simulink model "sm_backhoe"  (R2021b)
settings: Solver=ode23t  StartTime=0.0  StopTime=60  MaxStep=0.1  RelTol=1e-3  EnableMultiTasking=on
model workspace (MATLAB code in the model file):
  | cylinderGray = [0.6 0.6 0.6];
  | darkOrange = [0.8 0.5 0];
  | glassBlue = [0.2 0.2 1];
  | gray = [0.3 0.3 0.3];
  | orange = [0.8 0.65 0];
  | pistonGray = [0.4 0.4 0.4];
  | tireBlack = [0.1 0.1 0.1];
  | wheelGray = [0.6 0.6 0.6];
  | yellow = [0.8 0.8 0];
  | 
  | rhoGlass = 2500;
  | rhoRubber = 1500;
  | rhoSteel = 7800;
undefined symbols (not defined in the file): sigbuilder_block, X, Y, Z
libraries: sm_lib x161, sm_backhoe_lib x38, nesl_utility x9
(part 2 of 5)

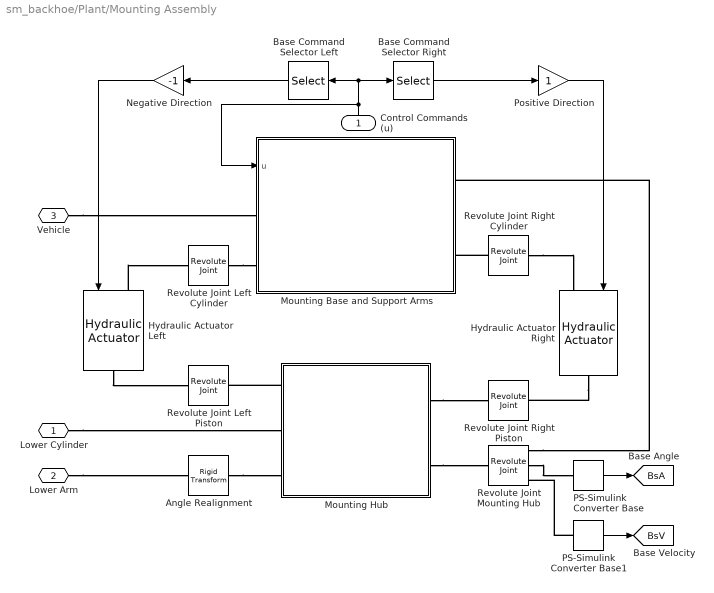
== system sm_backhoe/Plant/Mounting Assembly ==
  Control Commands (u) : Inport
  Angle Realignment : sm_lib/Frames and Transforms/Rigid Transform  TranslationMethod=None  TranslationStandardOffset=0.5  TranslationLengthUnit=m  TranslationStandardAxis=+Z  TranslationCartesianOffset=[ 0 0 0]  TranslationROffset=0  TranslationROffsetUnits=m  TranslationZOffset=0  TranslationZOffsetUnits=m  TranslationThetaOffset=0  TranslationThetaOffsetUnits=deg  RotationMethod=AlignedAxes  RotationAngleUnits=deg  RotationStandardAxis=-Z  RotationAngle=90  RotationArbitraryAxis=[0 0 1]  FollAlignAxisA=+Z  BaseAlignAxisA=+Z  FollAlignAxisB=+X  BaseAlignAxisB=-Y  RotationSequenceAxes=FollowerAxes  RotationSequence=XYX  RotationSequenceAngles=[0 0 0]  RotationSequenceAnglesUnits=deg  RotationMatrix=[1 0 0; 0 1 0; 0 0 1]
  Base Command Selector Left : Selector  InputPortWidth=5  IndexOptions=Index vector (dialog)  Indices=4  OutputSizes=1
  Base Command Selector Right : Selector  InputPortWidth=5  IndexOptions=Index vector (dialog)  Indices=4  OutputSizes=1
  Hydraulic Actuator Left : sm_backhoe_lib/Hydraulic Actuator  Lcyl=1.6  Rcyl=0.15  Lbase=0.65  Wbase=0.35  Rbp=0.075  Lbp=0.8  circlePointsCyl=25  circlePointsCylB=25  Lpist=1.75  Rpist=0.085  Whead=0.275  Lhead=0.5  Rhp=0.075  Lhp=0.9  circlePointsPist=25  cylColor=cylinderGray  rhoCyl=rhoSteel  pistColor=pistonGray  rhoPist=rhoSteel  connColor=gray  rhoConn=rhoSteel
      settings: SourceProductBaseCode=MS
  Hydraulic Actuator Right : sm_backhoe_lib/Hydraulic Actuator  Lcyl=1.6  Rcyl=0.15  Lbase=0.65  Wbase=0.35  Rbp=0.075  Lbp=0.8  circlePointsCyl=25  circlePointsCylB=25  Lpist=1.75  Rpist=0.085  Whead=0.275  Lhead=0.5  Rhp=0.075  Lhp=0.9  circlePointsPist=25  cylColor=cylinderGray  rhoCyl=rhoSteel  pistColor=pistonGray  rhoPist=rhoSteel  connColor=gray  rhoConn=rhoSteel
      settings: SourceProductBaseCode=MS
  Mounting Base and Support Arms : Subsystem
      mask Display:
      | image(fullfile(matlabroot,'toolbox','physmod','sm','smdemos','backhoe','images','sm_backhoe_mountingbaseassembly.png'));
      | port_label('input',1,'u');
      | port_label('lconn',1,'V');
      | port_label('lconn',2,'AL');
      | port_label('rconn',1,'MH');
      | port_label('rconn',2,'AR');
  Mounting Hub : Subsystem  mask(Mounting Hub){Hleft=1, Hright=2, Ltop=0.75, Lbottom=1.5, Tplate=0.3, Dplates=1.2, plateFillet=0.25, numPoints=15, L1=0.75, H1=0.25, RH1=0.075, L2=0.75, H2=1.75, RH2=0.075, L3=0.5, H3=0.5, Larm=0.8, Warm=0.5, Tarm=0.5, Tab=0.1, RH3=0.075, Dbracket=1.1, Lbracket=1.2, Wbracket=1.2, Tbracket=2, Hbracket=1, Rhole=0.1, Hhole=0.5, hubColor=orange, rho=rhoSteel}
      mask prompts: Hleft "Hleft (m)"; Hright "Hright (m)"; Ltop "Ltop (m)"; Lbottom "Lbottom (m)"; Tplate "Tplate (m)"; Dplates "Dplates (m)"; plateFillet "Plate Fillet Radius (m)"; numPoints "Fillet Resolution (pts/rev)"; L1 "L1 (m)"; H1 "H1 (m)"; RH1 "RH1 (m)"; L2 "L2 (m)"; H2 "H2 (m)"; RH2 "RH2 (m)"; L3 "L3 (m)"; H3 "H3 (m)"; Larm "Larm (m)"; Warm "Warm (m)"; Tarm "Tarm (m)"; Tab "Tab (m)"; RH3 "RH3 (m)"; Dbracket "Dbracket (m)"; Lbracket "Lbracket (m)"; Wbracket "Wbracket (m)"; Tbracket "Tbracket (m)"; Hbracket "Hbracket (m)"; Rhole "Rhole (m)"; Hhole "Hhole (m)"; hubColor "Hub Color"; rho "Density (kg/m^3)"
      mask help:
      | Consists of the backhoe mounting hub assembly.
      |
      | This assembly connects to the Backhoe Arm assembly on the front end, and to the Mounting Base assembly on the rear and side.
      |
      | Attachment points are:
      | LH: Left base hydraulic actuator (piston Head).
      | RH: Right base hydraulic actuator (piston Head).
      | LC: Lower arm hydraulic actuator (Cylinder base).
      | LA: Lower Arm joint.
      | MB: Mounting Base joint.
      | All attachments are configured for Revolute Joints.
      |
      | Click on Help to view a schematic of the bracket, its configurable dimension parameters and attachment points (in red).
      mask init:
      | plateSection = [0              0     ; ...
      |                 Lbottom        0     ; ...
      |                 Lbottom        Hright; ...
      |                 (Lbottom-Ltop) Hright; ...
      |                 0              Hleft];
      | plateSection = simmechanics.demohelpers.round_corners(plateSection,1:5,0.1,15);
      mask Help: web(fullfile(matlabroot,'toolbox','physmod','sm','smdemos','backhoe','demohelp','sm_backhoe_mountinghub.html'));
      mask Display:
      | image(fullfile(matlabroot,'toolbox','physmod','sm','smdemos','backhoe','images','sm_backhoe_mountinghub.png'));
      | port_label('lconn',1,'LH');
      | port_label('lconn',2,'LC');
      | port_label('lconn',3,'LA');
      | port_label('rconn',1,'RH');
      | port_label('rconn',2,'MB');
  Negative Direction : Gain  Gain=-1
  PS-Simulink Converter Base : nesl_utility/PS-Simulink Converter  PhysicalDomain=network_engine_domain  SubClassName=ps_output  LeftPortType=input  RightPortType=output  PseudoPeriodic=off  Frequencies=[]  Unit=deg  AffineConversion=off
      settings: SourceProductBaseCode=PW,SS
  PS-Simulink Converter Base1 : nesl_utility/PS-Simulink Converter  PhysicalDomain=network_engine_domain  SubClassName=ps_output  LeftPortType=input  RightPortType=output  PseudoPeriodic=off  Frequencies=[]  Unit=deg/s  AffineConversion=off
      settings: SourceProductBaseCode=PW,SS
  Positive Direction : Gain
  Revolute Joint Left Cylinder : sm_lib/Joints/Revolute Joint  JointMode=Normal  SenseConstraintForce=off  SenseConstraintForceX=off  SenseConstraintForceY=off  SenseConstraintForceZ=off  SenseConstraintTorque=off  SenseConstraintTorqueX=off  SenseConstraintTorqueY=off  SenseConstraintTorqueZ=off  SenseTotalForce=off  SenseTotalForceX=off  SenseTotalForceY=off  SenseTotalForceZ=off  SenseTotalTorque=off  SenseTotalTorqueX=off  SenseTotalTorqueY=off  SenseTotalTorqueZ=off  CompositeWrenchDir=FollowerOnBase  CompositeWrenchFrame=BaseFrame  EquilibriumPosition=0  EquilibriumPositionUnits=deg  SpringStiffness=0  SpringStiffnessUnits=N*m/deg  DampingCoefficient=0  DampingCoefficientUnits=N*m/(deg/s)  TorqueActuationMode=NoTorque  MotionActuationMode=ComputedMotion  SensePosition=off  SenseVelocity=off  SenseAcceleration=off  SenseTorqueForce=off  SenseLowerLimitTorqueForce=off  SenseUpperLimitTorqueForce=off  LowerLimitSpecify=off  LowerLimitBound=-90  LowerLimitBoundUnits=deg  LowerLimitStiffness=1e4  LowerLimitStiffnessUnits=N*m/deg  LowerLimitDamping=10  LowerLimitDampingUnits=N*m/(deg/s)  LowerLimitTransitionRegionWidth=0.1  LowerLimitTransitionRegionWidthUnits=deg  UpperLimitSpecify=off  UpperLimitBound=90  UpperLimitBoundUnits=deg  UpperLimitStiffness=1e4  UpperLimitStiffnessUnits=N*m/deg  UpperLimitDamping=10  UpperLimitDampingUnits=N*m/(deg/s)  UpperLimitTransitionRegionWidth=0.1  UpperLimitTransitionRegionWidthUnits=deg  PositionTargetSpecify=off  PositionTargetPriority=High  PositionTargetValue=0  PositionTargetValueUnits=deg  VelocityTargetSpecify=off  VelocityTargetPriority=High  VelocityTargetValue=0  VelocityTargetValueUnits=deg/s
  Revolute Joint Right Cylinder : sm_lib/Joints/Revolute Joint  JointMode=Normal  SenseConstraintForce=off  SenseConstraintForceX=off  SenseConstraintForceY=off  SenseConstraintForceZ=off  SenseConstraintTorque=off  SenseConstraintTorqueX=off  SenseConstraintTorqueY=off  SenseConstraintTorqueZ=off  SenseTotalForce=off  SenseTotalForceX=off  SenseTotalForceY=off  SenseTotalForceZ=off  SenseTotalTorque=off  SenseTotalTorqueX=off  SenseTotalTorqueY=off  SenseTotalTorqueZ=off  CompositeWrenchDir=FollowerOnBase  CompositeWrenchFrame=BaseFrame  EquilibriumPosition=0  EquilibriumPositionUnits=deg  SpringStiffness=0  SpringStiffnessUnits=N*m/deg  DampingCoefficient=0  DampingCoefficientUnits=N*m/(deg/s)  TorqueActuationMode=NoTorque  MotionActuationMode=ComputedMotion  SensePosition=off  SenseVelocity=off  SenseAcceleration=off  SenseTorqueForce=off  SenseLowerLimitTorqueForce=off  SenseUpperLimitTorqueForce=off  LowerLimitSpecify=off  LowerLimitBound=-90  LowerLimitBoundUnits=deg  LowerLimitStiffness=1e4  LowerLimitStiffnessUnits=N*m/deg  LowerLimitDamping=10  LowerLimitDampingUnits=N*m/(deg/s)  LowerLimitTransitionRegionWidth=0.1  LowerLimitTransitionRegionWidthUnits=deg  UpperLimitSpecify=off  UpperLimitBound=90  UpperLimitBoundUnits=deg  UpperLimitStiffness=1e4  UpperLimitStiffnessUnits=N*m/deg  UpperLimitDamping=10  UpperLimitDampingUnits=N*m/(deg/s)  UpperLimitTransitionRegionWidth=0.1  UpperLimitTransitionRegionWidthUnits=deg  PositionTargetSpecify=off  PositionTargetPriority=High  PositionTargetValue=0  PositionTargetValueUnits=deg  VelocityTargetSpecify=off  VelocityTargetPriority=High  VelocityTargetValue=0  VelocityTargetValueUnits=deg/s
  Revolute Joint Mounting Hub : sm_lib/Joints/Revolute Joint  JointMode=Normal  SenseConstraintForce=off  SenseConstraintForceX=off  SenseConstraintForceY=off  SenseConstraintForceZ=off  SenseConstraintTorque=off  SenseConstraintTorqueX=off  SenseConstraintTorqueY=off  SenseConstraintTorqueZ=off  SenseTotalForce=off  SenseTotalForceX=off  SenseTotalForceY=off  SenseTotalForceZ=off  SenseTotalTorque=off  SenseTotalTorqueX=off  SenseTotalTorqueY=off  SenseTotalTorqueZ=off  CompositeWrenchDir=FollowerOnBase  CompositeWrenchFrame=BaseFrame  EquilibriumPosition=0  EquilibriumPositionUnits=deg  SpringStiffness=1000  SpringStiffnessUnits=N*m/rad  DampingCoefficient=500  DampingCoefficientUnits=N*m/(rad/s)  TorqueActuationMode=NoTorque  MotionActuationMode=ComputedMotion  SensePosition=on  SenseVelocity=on  SenseAcceleration=off  SenseTorqueForce=off  SenseLowerLimitTorqueForce=off  SenseUpperLimitTorqueForce=off  LowerLimitSpecify=off  LowerLimitBound=-90  LowerLimitBoundUnits=deg  LowerLimitStiffness=1e4  LowerLimitStiffnessUnits=N*m/deg  LowerLimitDamping=10  LowerLimitDampingUnits=N*m/(deg/s)  LowerLimitTransitionRegionWidth=0.1  LowerLimitTransitionRegionWidthUnits=deg  UpperLimitSpecify=off  UpperLimitBound=90  UpperLimitBoundUnits=deg  UpperLimitStiffness=1e4  UpperLimitStiffnessUnits=N*m/deg  UpperLimitDamping=10  UpperLimitDampingUnits=N*m/(deg/s)  UpperLimitTransitionRegionWidth=0.1  UpperLimitTransitionRegionWidthUnits=deg  PositionTargetSpecify=on  PositionTargetPriority=Low  PositionTargetValue=0  PositionTargetValueUnits=deg  VelocityTargetSpecify=off  VelocityTargetPriority=High  VelocityTargetValue=0  VelocityTargetValueUnits=deg/s
  Revolute Joint Left Piston : sm_lib/Joints/Revolute Joint  JointMode=Normal  SenseConstraintForce=off  SenseConstraintForceX=off  SenseConstraintForceY=off  SenseConstraintForceZ=off  SenseConstraintTorque=off  SenseConstraintTorqueX=off  SenseConstraintTorqueY=off  SenseConstraintTorqueZ=off  SenseTotalForce=off  SenseTotalForceX=off  SenseTotalForceY=off  SenseTotalForceZ=off  SenseTotalTorque=off  SenseTotalTorqueX=off  SenseTotalTorqueY=off  SenseTotalTorqueZ=off  CompositeWrenchDir=FollowerOnBase  CompositeWrenchFrame=BaseFrame  EquilibriumPosition=0  EquilibriumPositionUnits=deg  SpringStiffness=0  SpringStiffnessUnits=N*m/deg  DampingCoefficient=0  DampingCoefficientUnits=N*m/(deg/s)  TorqueActuationMode=NoTorque  MotionActuationMode=ComputedMotion  SensePosition=off  SenseVelocity=off  SenseAcceleration=off  SenseTorqueForce=off  SenseLowerLimitTorqueForce=off  SenseUpperLimitTorqueForce=off  LowerLimitSpecify=off  LowerLimitBound=-90  LowerLimitBoundUnits=deg  LowerLimitStiffness=1e4  LowerLimitStiffnessUnits=N*m/deg  LowerLimitDamping=10  LowerLimitDampingUnits=N*m/(deg/s)  LowerLimitTransitionRegionWidth=0.1  LowerLimitTransitionRegionWidthUnits=deg  UpperLimitSpecify=off  UpperLimitBound=90  UpperLimitBoundUnits=deg  UpperLimitStiffness=1e4  UpperLimitStiffnessUnits=N*m/deg  UpperLimitDamping=10  UpperLimitDampingUnits=N*m/(deg/s)  UpperLimitTransitionRegionWidth=0.1  UpperLimitTransitionRegionWidthUnits=deg  PositionTargetSpecify=off  PositionTargetPriority=Low  PositionTargetValue=180  PositionTargetValueUnits=deg  VelocityTargetSpecify=off  VelocityTargetPriority=High  VelocityTargetValue=0  VelocityTargetValueUnits=deg/s
  Revolute Joint Right Piston : sm_lib/Joints/Revolute Joint  JointMode=Normal  SenseConstraintForce=off  SenseConstraintForceX=off  SenseConstraintForceY=off  SenseConstraintForceZ=off  SenseConstraintTorque=off  SenseConstraintTorqueX=off  SenseConstraintTorqueY=off  SenseConstraintTorqueZ=off  SenseTotalForce=off  SenseTotalForceX=off  SenseTotalForceY=off  SenseTotalForceZ=off  SenseTotalTorque=off  SenseTotalTorqueX=off  SenseTotalTorqueY=off  SenseTotalTorqueZ=off  CompositeWrenchDir=FollowerOnBase  CompositeWrenchFrame=BaseFrame  EquilibriumPosition=0  EquilibriumPositionUnits=deg  SpringStiffness=0  SpringStiffnessUnits=N*m/deg  DampingCoefficient=0  DampingCoefficientUnits=N*m/(deg/s)  TorqueActuationMode=NoTorque  MotionActuationMode=ComputedMotion  SensePosition=off  SenseVelocity=off  SenseAcceleration=off  SenseTorqueForce=off  SenseLowerLimitTorqueForce=off  SenseUpperLimitTorqueForce=off  LowerLimitSpecify=off  LowerLimitBound=-90  LowerLimitBoundUnits=deg  LowerLimitStiffness=1e4  LowerLimitStiffnessUnits=N*m/deg  LowerLimitDamping=10  LowerLimitDampingUnits=N*m/(deg/s)  LowerLimitTransitionRegionWidth=0.1  LowerLimitTransitionRegionWidthUnits=deg  UpperLimitSpecify=off  UpperLimitBound=90  UpperLimitBoundUnits=deg  UpperLimitStiffness=1e4  UpperLimitStiffnessUnits=N*m/deg  UpperLimitDamping=10  UpperLimitDampingUnits=N*m/(deg/s)  UpperLimitTransitionRegionWidth=0.1  UpperLimitTransitionRegionWidthUnits=deg  PositionTargetSpecify=off  PositionTargetPriority=Low  PositionTargetValue=0  PositionTargetValueUnits=deg  VelocityTargetSpecify=off  VelocityTargetPriority=High  VelocityTargetValue=0  VelocityTargetValueUnits=deg/s
  Lower Cylinder : PMIOPort  Side=Right
  Lower Arm : PMIOPort  Port=2  Side=Right
  Vehicle : PMIOPort  Port=3  Side=Left
  tag scope: BsA=global, BsV=global
  wires:
  Control Commands (u)/1 -> Base Command Selector Left/1, Base Command Selector Right/1, Mounting Base and Support Arms/1(u)
  PS-Simulink Converter Base/1 -> [BsA]
  Base Command Selector Left/1 -> Negative Direction/1
  Base Command Selector Right/1 -> Positive Direction/1
  Negative Direction/1 -> Hydraulic Actuator Left/1
  Positive Direction/1 -> Hydraulic Actuator Right/1
  PS-Simulink Converter Base1/1 -> [BsV]
  connections:
  Mounting Hub/RConn2 -- Revolute Joint Mounting Hub/LConn1
  Mounting Hub/LConn1 -- Revolute Joint Left Piston/RConn1
  Mounting Hub/RConn1 -- Revolute Joint Right Piston/RConn1
  Vehicle/RConn1 -- Mounting Base and Support Arms/LConn1
  Revolute Joint Mounting Hub/RConn1 -- Mounting Base and Support Arms/RConn1
  Revolute Joint Mounting Hub/RConn2 -- PS-Simulink Converter Base/LConn1
  Lower Arm/RConn1 -- Angle Realignment/RConn1
  Angle Realignment/LConn1 -- Mounting Hub/LConn3
  Revolute Joint Left Cylinder/LConn1 -- Mounting Base and Support Arms/LConn2
  Revolute Joint Right Cylinder/LConn1 -- Mounting Base and Support Arms/RConn2
  Revolute Joint Right Cylinder/RConn1 -- Hydraulic Actuator Right/LConn1
  Hydraulic Actuator Right/RConn1 -- Revolute Joint Right Piston/LConn1
  Hydraulic Actuator Left/RConn1 -- Revolute Joint Left Piston/LConn1
  Hydraulic Actuator Left/LConn1 -- Revolute Joint Left Cylinder/RConn1
  Lower Cylinder/RConn1 -- Mounting Hub/LConn2
  PS-Simulink Converter Base1/LConn1 -- Revolute Joint Mounting Hub/RConn3

== system sm_backhoe/Plant/Sensed Signals ==
  Vector Concatenate : Concatenate  NumInputs=10
  pv : Outport
  wires:
  [BuA] -> Vector Concatenate/1
  [SV] -> Vector Concatenate/10
  [SA] -> Vector Concatenate/9
  [BsV] -> Vector Concatenate/8
  [BsA] -> Vector Concatenate/7
  [LV] -> Vector Concatenate/6
  [LA] -> Vector Concatenate/5
  [UV] -> Vector Concatenate/4
  [UA] -> Vector Concatenate/3
  [BuV] -> Vector Concatenate/2
  Vector Concatenate/1 -> pv/1

== system sm_backhoe/Plant/Vehicle ==
  " Rear Right Wheel" : sm_backhoe_lib/Wheel  Rwheel=1  Rtire=1.75  Raxle=0.15  W=1.65  Nc=30  tireColor=tireBlack  rhoTire=rhoRubber  wheelColor=wheelGray  rhoWheel=rhoSteel
      settings: SourceProductBaseCode=MS
  Front Left Wheel : sm_backhoe_lib/Wheel  Rwheel=0.85  Rtire=1.5  Raxle=0.15  W=1.2  Nc=30  tireColor=tireBlack  rhoTire=rhoRubber  wheelColor=wheelGray  rhoWheel=rhoSteel
      settings: SourceProductBaseCode=MS
  Front Right Wheel : sm_backhoe_lib/Wheel  Rwheel=0.85  Rtire=1.5  Raxle=0.15  W=1.2  Nc=30  tireColor=tireBlack  rhoTire=rhoRubber  wheelColor=wheelGray  rhoWheel=rhoSteel
      settings: SourceProductBaseCode=MS
  Lower Vehicle : Subsystem  mask(Lower Vehicle){Wbody=3, Lbody=7.75, Hbody=2.25, Lfw=6, Hfw=0.5, Pfw=1.5, Lrw=1.85, Hrw=0.75, Prw=2, Raxle=0.15, color=yellow, rho=rhoSteel}
      mask prompts: Wbody "Wbody (m)"; Lbody "Lbody (m)"; Hbody "Hbody (m)"; Lfw "Lfw (m)"; Hfw "Hfw (m)"; Pfw "Pfw (m)"; Lrw "Lrw (m)"; Hrw "Hrw (m)"; Prw "Prw (m)"; Raxle "Raxle (m)"; color "Chassis Color"; rho "Density (kg/m^3)"
      mask help:
      | Consists of the backhoe lower vehicle assembly.
      |
      | Rigid attachment points are:
      | MA: Mounting Assembly.
      | UV: Upper Vehicle.
      |
      | Revolute joint attachment points are:
      | FLW: Front Left Wheel.
      | RLW: Rear Left Wheel.
      | FRW: Front Right Wheel.
      | RRW: Rear Right Wheel.
      |
      | Click on Help to view a schematic of the lower vehicle, its configurable dimension parameters and attachment points (in red).
      mask Help: web(fullfile(matlabroot,'toolbox','physmod','sm','smdemos','backhoe','demohelp','sm_backhoe_lowervehicle.html'));
      mask Display:
      | image(fullfile(matlabroot,'toolbox','physmod','sm','smdemos','backhoe','images','sm_backhoe_lowervehicle.png'));
      | port_label('rconn',1,'MA');
      | port_label('lconn',2,'RRW');
      | port_label('lconn',3,'FRW');
      | port_label('lconn',1,'UV');
      | port_label('rconn',2,'RLW');
      | port_label('rconn',3,'FLW');
  Rear Left Wheel : sm_backhoe_lib/Wheel  Rwheel=1  Rtire=1.75  Raxle=0.15  W=1.65  Nc=30  tireColor=tireBlack  rhoTire=rhoRubber  wheelColor=wheelGray  rhoWheel=rhoSteel
      settings: SourceProductBaseCode=MS
  Upper Vehicle : Subsystem  mask(Upper Vehicle){D=-0.25, L1=3.5, L2=2.5, L3=2, L4=1.5, H=4, W=2.75, T=0.2, Wroof=3.75, Lroof=4.4, Troof=0.4, Rfillet=0.75, numPoints=25, Hback=1.5, Wback=3, Lback=1.52, backFillet=1, roofColor=yellow, rhoRoof=rhoSteel, cageColor=gray, rhoCage=rhoSteel, windowColor=glassBlue, rhoWindow=rhoGlass, opacity=0.6, backColor=yellow, rhoBack=rhoSteel}
      mask prompts: D "D (m)"; L1 "L1 (m)"; L2 "L2 (m)"; L3 "L3 (m)"; L4 "L4 (m)"; H "H (m)"; W "W (m)"; T "T (m)"; Wroof "Wroof (m)"; Lroof "Lroof (m)"; Troof "Troof (m)"; Rfillet "Rfillet [m]"; numPoints "Fillet Point Resolution"; Hback "Hback (m)"; Wback "Wback (m)"; Lback "Lback (m)"; backFillet "backFillet (m)"; roofColor "Roof Color"; rhoRoof "Roof Density (kg/m^3)"; cageColor "Cage Color"; rhoCage "Cage Density (kg/m^3)"; windowColor "Window Color"; rhoWindow "Window Density (kg/m^3)"; opacity "Window Opacity"; backColor "Back Color"; rhoBack "Back Density (kg/m^3)"
      mask help:
      | Consists of the backhoe upper vehicle assembly. Components are the glass cage, the back and the roof of the backhoe model.
      |
      | There is one rigid attachment points to the Lower Vehicle (LV).
      |
      | Click on Help to view a schematic of the upper vehicle, its configurable dimension parameters and attachment points (in red).
      mask init:
      | fWindow = [-T/2          0.01 ; ...
      |            -T/2          H    ; ...
      |            -L3           H    ; ...
      |            -(L1-T/2)     0.01];
      |        
      | bWindow = [T/2          0.01 ; ...
      |            (L2-T/2)     0.01 ; ...
      |            L4           H    ; ...
      |            T/2          H   ];
      | 
      | roofSection = [ Wroof/2  Lroof/2; ...
      |                -Wroof/2  Lroof/2; ...
      |                -Wroof/2 -Lroof/2; ...
      |                 Wroof/2 -Lroof/2];
      | roofSection = simmechanics.demohelpers.round_corners(roofSection,1:4,Rfillet,numPoints);
      | 
      | theta = atan((L2-L4)/H);
      | 
      | backSection = [  0                     0    ; ...
      |                Lback                   0    ; ...
      |            (Lback-(Hback*sin(theta))) Hback ; ...
      |             -Hback*sin(theta)         Hback];
      | backSection = simmechanics.demohelpers.round_corners(backSection,3,backFillet,numPoints);
      mask Help: web(fullfile(matlabroot,'toolbox','physmod','sm','smdemos','backhoe','demohelp','sm_backhoe_uppervehicle.html'));
      mask Display:
      | image(fullfile(matlabroot,'toolbox','physmod','sm','smdemos','backhoe','images','sm_backhoe_uppervehicle.png'));
      | port_label('lconn',1,'LV');
  Mounting Assembly : PMIOPort  Side=Left
  Ground : PMIOPort  Port=2  Side=Right
  connections:
  Lower Vehicle/RConn1 -- Mounting Assembly/RConn1
  Lower Vehicle/LConn2 -- " Rear Right Wheel"/LConn1
  Lower Vehicle/LConn3 -- Front Right Wheel/LConn1
  Lower Vehicle/RConn3 -- Front Left Wheel/LConn1
  Lower Vehicle/RConn2 -- Rear Left Wheel/LConn1
  Lower Vehicle/LConn1 -- Ground/RConn1 -- Upper Vehicle/LConn1

== system sm_backhoe/Plant/Backhoe Arm/Bucket ==
  Arm Revolute Rotation : sm_lib/Frames and Transforms/Rigid Transform  TranslationMethod=None  TranslationStandardOffset=0  TranslationLengthUnit=m  TranslationStandardAxis=+X  TranslationCartesianOffset=[0 0 0]  TranslationROffset=0  TranslationROffsetUnits=m  TranslationZOffset=0  TranslationZOffsetUnits=m  TranslationThetaOffset=0  TranslationThetaOffsetUnits=deg  RotationMethod=AlignedAxes  RotationAngleUnits=deg  RotationStandardAxis=-Y  RotationAngle=180  RotationArbitraryAxis=[0 0 1]  FollAlignAxisA=+Y  BaseAlignAxisA=+Y  FollAlignAxisB=+X  BaseAlignAxisB=-X  RotationSequenceAxes=FollowerAxes  RotationSequence=XYX  RotationSequenceAngles=[0 0 0]  RotationSequenceAnglesUnits=deg  RotationMatrix=[1 0 0; 0 1 0; 0 0 1]
  Attachment Frame : Subsystem
      mask Display:
      | image(fullfile(matlabroot,'toolbox','physmod','sm','smdemos','backhoe','images','sm_backhoe_attach.png'));
      | port_label('lconn',1,'B');
      | port_label('rconn',1,'CA');
      | port_label('rconn',2,'UA');
  Bucket : Subsystem
      mask Display:
      | image(fullfile(matlabroot,'toolbox','physmod','sm','smdemos','backhoe','images','sm_backhoe_bucketcase.png'));
      | port_label('rconn',1,'AF');
  Crank Revolute Rotation : sm_lib/Frames and Transforms/Rigid Transform  TranslationMethod=None  TranslationStandardOffset=0  TranslationLengthUnit=m  TranslationStandardAxis=+X  TranslationCartesianOffset=[0 0 0]  TranslationROffset=0  TranslationROffsetUnits=m  TranslationZOffset=0  TranslationZOffsetUnits=m  TranslationThetaOffset=0  TranslationThetaOffsetUnits=deg  RotationMethod=AlignedAxes  RotationAngleUnits=deg  RotationStandardAxis=-Y  RotationAngle=180  RotationArbitraryAxis=[0 0 1]  FollAlignAxisA=+Y  BaseAlignAxisA=+Y  FollAlignAxisB=+X  BaseAlignAxisB=-X  RotationSequenceAxes=FollowerAxes  RotationSequence=XYX  RotationSequenceAngles=[0 0 0]  RotationSequenceAnglesUnits=deg  RotationMatrix=[1 0 0; 0 1 0; 0 0 1]
  Crank Arm : PMIOPort  Side=Right
  Upper Arm : PMIOPort  Port=2  Side=Right
  connections:
  Bucket/RConn1 -- Attachment Frame/LConn1
  Crank Revolute Rotation/LConn1 -- Attachment Frame/RConn1
  Arm Revolute Rotation/LConn1 -- Attachment Frame/RConn2
  Upper Arm/RConn1 -- Arm Revolute Rotation/RConn1
  Crank Arm/RConn1 -- Crank Revolute Rotation/RConn1

== system sm_backhoe/Plant/Backhoe Arm/Lower Arm Assembly ==
  Angle Rotation : sm_lib/Frames and Transforms/Rigid Transform  TranslationMethod=None  TranslationStandardOffset=0  TranslationLengthUnit=m  TranslationStandardAxis=+Z  TranslationCartesianOffset=[0 0 0]  TranslationROffset=0  TranslationROffsetUnits=m  TranslationZOffset=0  TranslationZOffsetUnits=m  TranslationThetaOffset=0  TranslationThetaOffsetUnits=deg  RotationMethod=AlignedAxes  RotationAngleUnits=deg  RotationStandardAxis=+Z  RotationAngle=180  RotationArbitraryAxis=[0 0 1]  FollAlignAxisA=+Z  BaseAlignAxisA=+Z  FollAlignAxisB=+Y  BaseAlignAxisB=-Y  RotationSequenceAxes=FollowerAxes  RotationSequence=XYX  RotationSequenceAngles=[0 0 0]  RotationSequenceAnglesUnits=deg  RotationMatrix=[1 0 0; 0 1 0; 0 0 1]
  Bracket Double Hole : sm_backhoe_lib/Bracket Double Hole  Hbracket=0.75  Wbracket=1.5  Tbracket=0.15  Dbracket=0.75  Hhole=0.5  Dhole=0.75  Rhole=0.075  Rfillet=0.375  Nc=25  bracketColor=orange  rho=rhoSteel
      settings: SourceProductBaseCode=MS
  Front Bracket : sm_backhoe_lib/Bracket  Hbracket=0.65  Wbracket=0.5  Tbracket=0.225  Dbracket=0.45  Hhole=0.4  Rhole=0.075  circlePoints=25  bracketColor=darkOrange  rho=rhoSteel
      settings: SourceProductBaseCode=MS
  Lower Arm : Subsystem  mask(Lower Arm){Lbar=7, Wbar=0.8, Tbar=0.85, Lb=0.5, barFillet=0.1, numPoints=15, armColor=yellow, rho=rhoSteel}
      mask prompts: Lbar "Lbar (m)"; Wbar "Wbar (m)"; Tbar "Tbar (m)"; Lb "Lb (m)"; barFillet "Bar Fillet Radius (m)"; numPoints "Fillet Resolution (pts/rev)"; armColor "Arm Color"; rho "Density (kg/m^3)"
      mask help:
      | Consists of the backhoe lower arm and three attachment brackets -- front, rear and upper
      |
      | Attachment Points are:
      | MA: Mounting Assembly attachment.
      | LH: Lower arm hydraulic actuator (piston Head).
      | UA: Upper arm attachment.
      | UC: Upper arm hydraulic actuator (Cylinder base).
      | All attachments are configured for Revolute joints.
      |
      | The length Lb corresponds to the lengths measured from the center of the bar to the center of the upper bracket.
      |
      | The front and rear brackets are automatically placed at the center of the end faces of the upper arm bar.
      |
      | Click on Help to view a schematic of the lower arm, its configurable dimension parameters and attachment points (in red).
      mask init:
      | barSection = [Tbar/2 Wbar/2;  ...
      |              -Tbar/2 Wbar/2;  ...
      |              -Tbar/2 -Wbar/2; ...
      |               Tbar/2 -Wbar/2];
      | barSection = simmechanics.demohelpers.round_corners(barSection,1:4,barFillet,numPoints);
      mask Help: web(fullfile(matlabroot,'toolbox','physmod','sm','smdemos','backhoe','demohelp','sm_backhoe_lowerarm.html'));
      mask Display:
      | image(fullfile(matlabroot,'toolbox','physmod','sm','smdemos','backhoe','images','sm_backhoe_lowerarm.png'));
      | port_label('rconn',1,'RB');
      | port_label('lconn',2,'FB');;
      | port_label('lconn',1,'UB');
  Pin : sm_lib/Body Elements/Cylindrical Solid  GraphicAmbientColor=[0.15 0.15 0.15 1.0]  BasedOnType=Density  CenterOfMass=[0 0 0]  CenterOfMassUnits=m  GraphicDiffuseColor=gray  CylinderLength=0.8  CylinderLengthUnits=m  CylinderRadius=0.075  CylinderRadiusUnits=m  Density=rhoSteel  DensityUnits=kg/(m^3)  DoExposeReferenceFrame=on  GraphicEmissiveColor=[0.0 0.0 0.0 1.0]  ExportEntireGeometry=off  SerializedFrames=<Frames/>  MarkerShape=Sphere  MarkerSize=10  GraphicType=FromGeometry  InertiaType=CalculateFromGeometry  Mass=1  MassUnits=kg  MomentsOfInertia=[1 1 1]  MomentsOfInertiaUnits=kg*m^2  GraphicOpacity=1.0  ProductsOfInertia=[0 0 0]  ProductsOfInertiaUnits=kg*m^2  GraphicShininess=75  GraphicSpecularColor=[0.5 0.5 0.5 1.0]  GraphicVisPropType=SimpleVisualProperties
  Pin1 : sm_lib/Body Elements/Cylindrical Solid  GraphicAmbientColor=[0.15 0.15 0.15 1.0]  BasedOnType=Density  CenterOfMass=[0 0 0]  CenterOfMassUnits=m  GraphicDiffuseColor=gray  CylinderLength=0.8  CylinderLengthUnits=m  CylinderRadius=0.075  CylinderRadiusUnits=m  Density=rhoSteel  DensityUnits=kg/(m^3)  DoExposeReferenceFrame=on  GraphicEmissiveColor=[0.0 0.0 0.0 1.0]  ExportEntireGeometry=off  SerializedFrames=<Frames/>  MarkerShape=Sphere  MarkerSize=10  GraphicType=FromGeometry  InertiaType=CalculateFromGeometry  Mass=1  MassUnits=kg  MomentsOfInertia=[1 1 1]  MomentsOfInertiaUnits=kg*m^2  GraphicOpacity=1.0  ProductsOfInertia=[0 0 0]  ProductsOfInertiaUnits=kg*m^2  GraphicShininess=75  GraphicSpecularColor=[0.5 0.5 0.5 1.0]  GraphicVisPropType=SimpleVisualProperties
  Pin2 : sm_lib/Body Elements/Cylindrical Solid  GraphicAmbientColor=[0.15 0.15 0.15 1.0]  BasedOnType=Density  CenterOfMass=[0 0 0]  CenterOfMassUnits=m  GraphicDiffuseColor=gray  CylinderLength=0.8  CylinderLengthUnits=m  CylinderRadius=0.075  CylinderRadiusUnits=m  Density=rhoSteel  DensityUnits=kg/(m^3)  DoExposeReferenceFrame=on  GraphicEmissiveColor=[0.0 0.0 0.0 1.0]  ExportEntireGeometry=off  SerializedFrames=<Frames/>  MarkerShape=Sphere  MarkerSize=10  GraphicType=FromGeometry  InertiaType=CalculateFromGeometry  Mass=1  MassUnits=kg  MomentsOfInertia=[1 1 1]  MomentsOfInertiaUnits=kg*m^2  GraphicOpacity=1.0  ProductsOfInertia=[0 0 0]  ProductsOfInertiaUnits=kg*m^2  GraphicShininess=75  GraphicSpecularColor=[0.5 0.5 0.5 1.0]  GraphicVisPropType=SimpleVisualProperties
  Rear Bracket : sm_backhoe_lib/Bracket  Hbracket=0.75  Wbracket=0.75  Tbracket=0.15  Dbracket=0.75  Hhole=0.5  Rhole=0.075  circlePoints=25  bracketColor=darkOrange  rho=rhoSteel
      settings: SourceProductBaseCode=MS
  Lower Head : PMIOPort  Side=Left
  Mounting Assembly : PMIOPort  Port=2  Side=Left
  Upper Cylinder : PMIOPort  Port=3  Side=Right
  Upper Arm : PMIOPort  Port=4  Side=Right
  connections:
  Mounting Assembly/RConn1 -- Rear Bracket/RConn1
  Lower Arm/RConn1 -- Rear Bracket/LConn1
  Front Bracket/RConn1 -- Pin/RConn1 -- Angle Rotation/LConn1
  Front Bracket/LConn1 -- Lower Arm/LConn2
  Upper Arm/RConn1 -- Angle Rotation/RConn1
  Lower Arm/LConn1 -- Bracket Double Hole/LConn1
  Lower Head/RConn1 -- Bracket Double Hole/RConn2 -- Pin1/RConn1
  Pin2/RConn1 -- Bracket Double Hole/RConn1 -- Upper Cylinder/RConn1

== system sm_backhoe/Plant/Backhoe Arm/Upper Arm Assembly ==
  Pressure [Bucket Joint] : Inport
  Angle Realignment : sm_lib/Frames and Transforms/Rigid Transform  TranslationMethod=None  TranslationStandardOffset=0  TranslationLengthUnit=m  TranslationStandardAxis=+Z  TranslationCartesianOffset=[0 0 0]  TranslationROffset=0  TranslationROffsetUnits=m  TranslationZOffset=0  TranslationZOffsetUnits=m  TranslationThetaOffset=0  TranslationThetaOffsetUnits=deg  RotationMethod=AlignedAxes  RotationAngleUnits=deg  RotationStandardAxis=-Z  RotationAngle=90  RotationArbitraryAxis=[0 0 1]  FollAlignAxisA=+X  BaseAlignAxisA=-Y  FollAlignAxisB=+Z  BaseAlignAxisB=+Z  RotationSequenceAxes=FollowerAxes  RotationSequence=XYX  RotationSequenceAngles=[0 0 0]  RotationSequenceAnglesUnits=deg  RotationMatrix=[1 0 0; 0 1 0; 0 0 1]
  Arm-Actuator Joint : sm_lib/Joints/Revolute Joint  JointMode=Normal  SenseConstraintForce=off  SenseConstraintForceX=off  SenseConstraintForceY=off  SenseConstraintForceZ=off  SenseConstraintTorque=off  SenseConstraintTorqueX=off  SenseConstraintTorqueY=off  SenseConstraintTorqueZ=off  SenseTotalForce=off  SenseTotalForceX=off  SenseTotalForceY=off  SenseTotalForceZ=off  SenseTotalTorque=off  SenseTotalTorqueX=off  SenseTotalTorqueY=off  SenseTotalTorqueZ=off  CompositeWrenchDir=FollowerOnBase  CompositeWrenchFrame=BaseFrame  EquilibriumPosition=0  EquilibriumPositionUnits=deg  SpringStiffness=0  SpringStiffnessUnits=N*m/deg  DampingCoefficient=0  DampingCoefficientUnits=N*m/(deg/s)  TorqueActuationMode=NoTorque  MotionActuationMode=ComputedMotion  SensePosition=off  SenseVelocity=off  SenseAcceleration=off  SenseTorqueForce=off  SenseLowerLimitTorqueForce=off  SenseUpperLimitTorqueForce=off  LowerLimitSpecify=off  LowerLimitBound=-90  LowerLimitBoundUnits=deg  LowerLimitStiffness=1e4  LowerLimitStiffnessUnits=N*m/deg  LowerLimitDamping=10  LowerLimitDampingUnits=N*m/(deg/s)  LowerLimitTransitionRegionWidth=0.1  LowerLimitTransitionRegionWidthUnits=deg  UpperLimitSpecify=off  UpperLimitBound=90  UpperLimitBoundUnits=deg  UpperLimitStiffness=1e4  UpperLimitStiffnessUnits=N*m/deg  UpperLimitDamping=10  UpperLimitDampingUnits=N*m/(deg/s)  UpperLimitTransitionRegionWidth=0.1  UpperLimitTransitionRegionWidthUnits=deg  PositionTargetSpecify=on  PositionTargetPriority=Low  PositionTargetValue=-90  PositionTargetValueUnits=deg  VelocityTargetSpecify=off  VelocityTargetPriority=High  VelocityTargetValue=0  VelocityTargetValueUnits=deg/s
  Crank-Actuator Joint : sm_lib/Joints/Revolute Joint  JointMode=Normal  SenseConstraintForce=off  SenseConstraintForceX=off  SenseConstraintForceY=off  SenseConstraintForceZ=off  SenseConstraintTorque=off  SenseConstraintTorqueX=off  SenseConstraintTorqueY=off  SenseConstraintTorqueZ=off  SenseTotalForce=off  SenseTotalForceX=off  SenseTotalForceY=off  SenseTotalForceZ=off  SenseTotalTorque=off  SenseTotalTorqueX=off  SenseTotalTorqueY=off  SenseTotalTorqueZ=off  CompositeWrenchDir=FollowerOnBase  CompositeWrenchFrame=BaseFrame  EquilibriumPosition=0  EquilibriumPositionUnits=deg  SpringStiffness=0  SpringStiffnessUnits=N*m/deg  DampingCoefficient=0  DampingCoefficientUnits=N*m/(deg/s)  TorqueActuationMode=NoTorque  MotionActuationMode=ComputedMotion  SensePosition=off  SenseVelocity=off  SenseAcceleration=off  SenseTorqueForce=off  SenseLowerLimitTorqueForce=off  SenseUpperLimitTorqueForce=off  LowerLimitSpecify=off  LowerLimitBound=-90  LowerLimitBoundUnits=deg  LowerLimitStiffness=1e4  LowerLimitStiffnessUnits=N*m/deg  LowerLimitDamping=10  LowerLimitDampingUnits=N*m/(deg/s)  LowerLimitTransitionRegionWidth=0.1  LowerLimitTransitionRegionWidthUnits=deg  UpperLimitSpecify=off  UpperLimitBound=90  UpperLimitBoundUnits=deg  UpperLimitStiffness=1e4  UpperLimitStiffnessUnits=N*m/deg  UpperLimitDamping=10  UpperLimitDampingUnits=N*m/(deg/s)  UpperLimitTransitionRegionWidth=0.1  UpperLimitTransitionRegionWidthUnits=deg  PositionTargetSpecify=off  PositionTargetPriority=High  PositionTargetValue=0  PositionTargetValueUnits=deg  VelocityTargetSpecify=off  VelocityTargetPriority=High  VelocityTargetValue=0  VelocityTargetValueUnits=deg/s
  Hydraulic Actuator Upper Arm - Bucket : sm_backhoe_lib/Hydraulic Actuator  Lcyl=1.9  Rcyl=0.2  Lbase=0.65  Wbase=0.425  Rbp=0.075  Lbp=0.8  circlePointsCyl=25  circlePointsCylB=25  Lpist=1.9  Rpist=0.12  Whead=0.35  Lhead=0.65  Rhp=0.075  Lhp=0.9  circlePointsPist=25  cylColor=cylinderGray  rhoCyl=rhoSteel  pistColor=pistonGray  rhoPist=rhoSteel  connColor=gray  rhoConn=rhoSteel
      settings: SourceProductBaseCode=MS
  Upper Arm and Crank : Subsystem
      mask Display:
      | image(fullfile(matlabroot,'toolbox','physmod','sm','smdemos','backhoe','images','sm_backhoe_upperassembly.png'));
      | port_label('lconn',1,'CB');
      | port_label('lconn',2,'UH');
      | port_label('lconn',3,'LA');
      | port_label('rconn',1,'BA');
      | port_label('rconn',2,'BC');
      | port_label('rconn',3,'BH');
  Upper Head : PMIOPort  Side=Left
  Lower Arm : PMIOPort  Port=2  Side=Left
  Crank Arm : PMIOPort  Port=3  Side=Right
  Bucket : PMIOPort  Port=4  Side=Right
  wires:
  Pressure [Bucket Joint]/1 -> Hydraulic Actuator Upper Arm - Bucket/1
  connections:
  Angle Realignment/RConn1 -- Bucket/RConn1
  Hydraulic Actuator Upper Arm - Bucket/LConn1 -- Arm-Actuator Joint/RConn1
  Crank-Actuator Joint/LConn1 -- Hydraulic Actuator Upper Arm - Bucket/RConn1
  Lower Arm/RConn1 -- Upper Arm and Crank/LConn3
  Arm-Actuator Joint/LConn1 -- Upper Arm and Crank/LConn1
  Crank-Actuator Joint/RConn1 -- Upper Arm and Crank/RConn1
  Crank Arm/RConn1 -- Upper Arm and Crank/RConn2
  Angle Realignment/LConn1 -- Upper Arm and Crank/RConn3
  Upper Head/RConn1 -- Upper Arm and Crank/LConn2

== system sm_backhoe/Plant/Mounting Assembly/Mounting Base and Support Arms ==
  u : Inport
  Bracket Assembly : Subsystem  mask(Bracket Assembly){Dbracket=2.75, Tbracket=0.35, Wbracket=1.5, Hbracket=1.35, Hhole=0.9, Rhole=0.1, Thub=0.25, Lweb=1.25, Hweb=2.4, bracketColor=darkOrange, webColor=darkOrange, rho=rhoSteel}
      mask prompts: Dbracket "Dbracket (m)"; Tbracket "Tbracket (m)"; Wbracket "Wbracket (m)"; Hbracket "Hbracket (m)"; Hhole "Hhole (m)"; Rhole "Rhole (m)"; Thub "Thub (m)"; Lweb "Lweb (m)"; Hweb "Hweb (m)"; bracketColor "Bracket Color"; webColor "Web Color"; rho "Density (kg/m^3)"
      mask help:
      | Consists of the backhoe mounting base bracket assembly.
      |
      | Attachment points are:
      | MB: Mounting Base, which is a rigid connection.
      | MH: Mounting Hub, which is configured for a Revolute joint.
      |
      | Click on Help to view a schematic of the bracket assembly, its configurable dimension parameters and attachment points (in red).
      mask Help: web(fullfile(matlabroot,'toolbox','physmod','sm','smdemos','backhoe','demohelp','sm_backhoe_bracketassembly.html'));
      mask Display:
      | image(fullfile(matlabroot,'toolbox','physmod','sm','smdemos','backhoe','images','sm_backhoe_bracketassembly.png'));
      | port_label('lconn',1,'MH');
      | port_label('rconn',1,'MB');
  Mounting Base : Subsystem  mask(Mounting Base){Lbase=4, Wbase=1.5, Wside=1.5, Lside=2.25, T=0.35, Hbracket=0.75, Wbracket=0.75, Tbracket=0.15, Dbracket=0.7, Hhole=0.5, Rhole=0.075, H=0.75, D=1.1, baseColor=yellow, bracketColor=orange, rho=rhoSteel, circlePoints=25}
      mask prompts: Lbase "Lbase (m)"; Wbase "Wbase (m)"; Wside "Wside (m)"; Lside "Lside (m)"; T "T (m)"; Hbracket "Hbracket (m)"; Wbracket "Wbracket (m)"; Tbracket "Tbracket (m)"; Dbracket "Dbracket (m)"; Hhole "Hhole (m)"; Rhole "Rhole (m)"; H "H (m)"; D "D (m)"; baseColor "Base Color"; bracketColor "Piston Bracket Color"; rho "Density (kg/m^3)"; circlePoints "Circle Resolution (pts/rev)"
      mask help:
      | Consists of the backhoe mounting base assembly.
      |
      | Rigid attachment points are:
      | BA: Bracket Assembly.
      | V: Vehicle.
      | LB: Left Bracket for support arms.
      | RB: Right Bracket for support arms.
      |
      | Revolute joint attachment points are:
      | LC: Left Cylinder base for base hydraulic actuator.
      | RC: Right Cylinder base for base hydraulic actuator.
      |
      | Click on Help to view a schematic of the mounting base, its configurable dimension parameters and attachment points (in red).
      mask Help: web(fullfile(matlabroot,'toolbox','physmod','sm','smdemos','backhoe','demohelp','sm_backhoe_mountingbase.html'));
      mask Display:
      | image(fullfile(matlabroot,'toolbox','physmod','sm','smdemos','backhoe','images','sm_backhoe_mountingbase.png'));
      | port_label('lconn',1,'BA');
      | port_label('lconn',2,'LB');
      | port_label('lconn',3,'LC');
      | port_label('rconn',1,'V');
      | port_label('rconn',2,'RB');
      | port_label('rconn',3,'RC');
  Support Arm Cmd Selector : Selector  InputPortWidth=5  IndexOptions=Index vector (dialog)  Indices=5  OutputSizes=1
  Support Arm Left : sm_backhoe_lib/Support Arm Assembly  Hbracket=0.8  Wbracket=1.75  Tbracket=0.15  Dbracket=0.8  HShoulderHole=0.5  DShoulderHole=1  RShoulderHole=0.075  RShoulderFillet=0.4  Larm=2.5  Warm=0.5  Tarm=0.35  Dhole=2  Rhole=0.075  AFAngle=45  Lpin=0.85  Lfoot=2  Wfoot=1  Tfoot=0.2  Dconn=1  Hhole=0.3  Rfillet=0.4  Lcyl=1.35  Rcyl=0.2  Lbase=0.65  Wbase=0.425  Rbp=0.075  Lbp=0.8  Lpist=1.35  Rpist=0.1  Lhead=0.5  Whead=0.275  Rhp=0.075  Lhp=0.8  circlePointsPist=25  circlePointsCyl=25  circlePointsCylB=25  circlePointsShoulder=25  circlePointsArm=25  circlePointsFoot=25  shoulderColor=orange  armColor=yellow  bracketColor=orange  footColor=yellow  pinColor=gray  pistonGray=pistonGray  cylinderGray=cylinderGray  rho=rhoSteel
      settings: SourceProductBaseCode=MS
  Support Arm Right : sm_backhoe_lib/Support Arm Assembly  Hbracket=0.8  Wbracket=1.75  Tbracket=0.15  Dbracket=0.8  HShoulderHole=0.5  DShoulderHole=1  RShoulderHole=0.075  RShoulderFillet=0.4  Larm=2.5  Warm=0.5  Tarm=0.35  Dhole=2  Rhole=0.075  AFAngle=45  Lpin=0.85  Lfoot=2  Wfoot=1  Tfoot=0.2  Dconn=1  Hhole=0.3  Rfillet=0.4  Lcyl=1.35  Rcyl=0.2  Lbase=0.65  Wbase=0.425  Rbp=0.075  Lbp=0.8  Lpist=1.35  Rpist=0.1  Lhead=0.5  Whead=0.275  Rhp=0.075  Lhp=0.8  circlePointsPist=25  circlePointsCyl=25  circlePointsCylB=25  circlePointsShoulder=25  circlePointsArm=25  circlePointsFoot=25  shoulderColor=orange  armColor=yellow  bracketColor=orange  footColor=yellow  pinColor=gray  pistonGray=pistonGray  cylinderGray=cylinderGray  rho=rhoSteel
      settings: SourceProductBaseCode=MS
  Terminator : Terminator
  Terminator1 : Terminator
  Mounting Hub : PMIOPort  Side=Right
  Vehicle : PMIOPort  Port=2  Side=Left
  Left Cylinder : PMIOPort  Port=3  Side=Left
  Right Cylinder : PMIOPort  Port=4  Side=Right
  tag scope: SA=global, SV=global
  wires:
  u/1 -> Support Arm Cmd Selector/1
  Support Arm Right/1 -> Terminator/1
  Support Arm Left/1 -> [SA]
  Support Arm Cmd Selector/1 -> Support Arm Right/1, Support Arm Left/1
  Support Arm Right/2 -> Terminator1/1
  Support Arm Left/2 -> [SV]
  connections:
  Mounting Hub/RConn1 -- Bracket Assembly/LConn1
  Vehicle/RConn1 -- Mounting Base/RConn1
  Bracket Assembly/RConn1 -- Mounting Base/LConn1
  Left Cylinder/RConn1 -- Mounting Base/LConn2
  Mounting Base/RConn2 -- Right Cylinder/RConn1
  Support Arm Left/LConn1 -- Mounting Base/LConn3
  Mounting Base/RConn3 -- Support Arm Right/LConn1

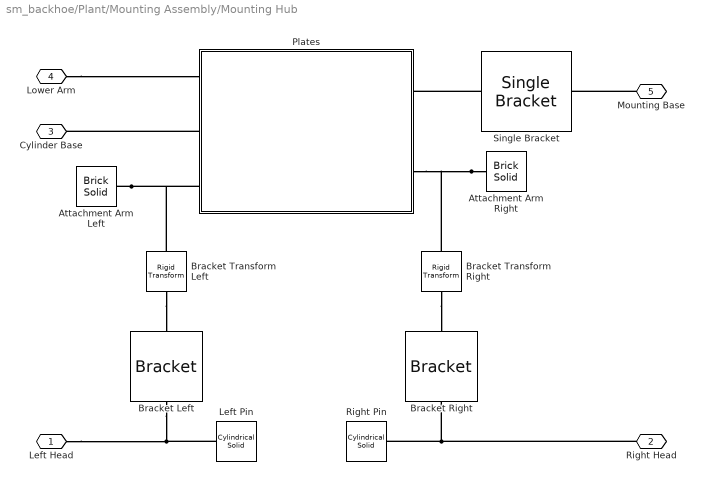
== system sm_backhoe/Plant/Mounting Assembly/Mounting Hub ==
  Attachment Arm Left : sm_lib/Body Elements/Brick Solid  GraphicAmbientColor=[0.15 0.15 0.15 1.0]  BasedOnType=Density  BrickDimensions=[Warm Tarm (Larm-Warm)]  BrickDimensionUnits=m  CenterOfMass=[0 0 0]  CenterOfMassUnits=m  GraphicDiffuseColor=hubColor  Density=rho  DensityUnits=kg/(m^3)  DoExposeReferenceFrame=on  GraphicEmissiveColor=[0.0 0.0 0.0 1.0]  ExportEntireGeometry=off  SerializedFrames=<Frames/>  MarkerShape=Sphere  MarkerSize=10  GraphicType=FromGeometry  InertiaType=CalculateFromGeometry  Mass=1  MassUnits=kg  MomentsOfInertia=[1 1 1]  MomentsOfInertiaUnits=kg*m^2  GraphicOpacity=1.0  ProductsOfInertia=[0 0 0]  ProductsOfInertiaUnits=kg*m^2  GraphicShininess=75  GraphicSpecularColor=[0.5 0.5 0.5 1.0]  GraphicVisPropType=SimpleVisualProperties
  Attachment Arm Right : sm_lib/Body Elements/Brick Solid  GraphicAmbientColor=[0.15 0.15 0.15 1.0]  BasedOnType=Density  BrickDimensions=[Warm Tarm (Larm-Warm)]  BrickDimensionUnits=m  CenterOfMass=[0 0 0]  CenterOfMassUnits=m  GraphicDiffuseColor=hubColor  Density=rho  DensityUnits=kg/(m^3)  DoExposeReferenceFrame=on  GraphicEmissiveColor=[0.0 0.0 0.0 1.0]  ExportEntireGeometry=off  SerializedFrames=<Frames/>  MarkerShape=Sphere  MarkerSize=10  GraphicType=FromGeometry  InertiaType=CalculateFromGeometry  Mass=1  MassUnits=kg  MomentsOfInertia=[1 1 1]  MomentsOfInertiaUnits=kg*m^2  GraphicOpacity=1.0  ProductsOfInertia=[0 0 0]  ProductsOfInertiaUnits=kg*m^2  GraphicShininess=75  GraphicSpecularColor=[0.5 0.5 0.5 1.0]  GraphicVisPropType=SimpleVisualProperties
  Bracket Transform Left : sm_lib/Frames and Transforms/Rigid Transform  TranslationMethod=StandardAxis  TranslationStandardOffset=(Larm-Warm)/2  TranslationLengthUnit=m  TranslationStandardAxis=+Z  TranslationCartesianOffset=[0 0 0]  TranslationROffset=0  TranslationROffsetUnits=m  TranslationZOffset=0  TranslationZOffsetUnits=m  TranslationThetaOffset=0  TranslationThetaOffsetUnits=deg  RotationMethod=AlignedAxes  RotationAngleUnits=deg  RotationStandardAxis=+Y  RotationAngle=180  RotationArbitraryAxis=[0 0 1]  FollAlignAxisA=+Z  BaseAlignAxisA=+Z  FollAlignAxisB=+X  BaseAlignAxisB=+X  RotationSequenceAxes=FollowerAxes  RotationSequence=XYX  RotationSequenceAngles=[0 0 0]  RotationSequenceAnglesUnits=deg  RotationMatrix=[1 0 0; 0 1 0; 0 0 1]
  Bracket Transform Right : sm_lib/Frames and Transforms/Rigid Transform  TranslationMethod=StandardAxis  TranslationStandardOffset=(Larm-Warm)/2  TranslationLengthUnit=m  TranslationStandardAxis=-Z  TranslationCartesianOffset=[0 0 0]  TranslationROffset=0  TranslationROffsetUnits=m  TranslationZOffset=0  TranslationZOffsetUnits=m  TranslationThetaOffset=0  TranslationThetaOffsetUnits=deg  RotationMethod=AlignedAxes  RotationAngleUnits=deg  RotationStandardAxis=+Y  RotationAngle=180  RotationArbitraryAxis=[0 0 1]  FollAlignAxisA=+Z  BaseAlignAxisA=-Z  FollAlignAxisB=+Y  BaseAlignAxisB=+Y  RotationSequenceAxes=FollowerAxes  RotationSequence=XYX  RotationSequenceAngles=[0 0 0]  RotationSequenceAnglesUnits=deg  RotationMatrix=[1 0 0; 0 1 0; 0 0 1]
  Bracket Left : sm_backhoe_lib/Bracket  Hbracket=Warm  Wbracket=Warm  Tbracket=Tab  Dbracket=Tarm  Hhole=Warm/2  Rhole=RH3  circlePoints=25  bracketColor=hubColor  rho=rho
      settings: SourceProductBaseCode=MS
  Bracket Right : sm_backhoe_lib/Bracket  Hbracket=Warm  Wbracket=Warm  Tbracket=Tab  Dbracket=Tarm  Hhole=Warm/2  Rhole=RH3  circlePoints=25  bracketColor=hubColor  rho=rho
      settings: SourceProductBaseCode=MS
  Left Pin : sm_lib/Body Elements/Cylindrical Solid  GraphicAmbientColor=[0.15 0.15 0.15 1.0]  BasedOnType=Density  CenterOfMass=[0 0 0]  CenterOfMassUnits=m  GraphicDiffuseColor=gray  CylinderLength=Tarm*1.2  CylinderLengthUnits=m  CylinderRadius=RH3  CylinderRadiusUnits=m  Density=rhoSteel  DensityUnits=kg/(m^3)  DoExposeReferenceFrame=on  GraphicEmissiveColor=[0.0 0.0 0.0 1.0]  ExportEntireGeometry=off  SerializedFrames=<Frames/>  MarkerShape=Sphere  MarkerSize=10  GraphicType=FromGeometry  InertiaType=CalculateFromGeometry  Mass=1  MassUnits=kg  MomentsOfInertia=[1 1 1]  MomentsOfInertiaUnits=kg*m^2  GraphicOpacity=1.0  ProductsOfInertia=[0 0 0]  ProductsOfInertiaUnits=kg*m^2  GraphicShininess=75  GraphicSpecularColor=[0.5 0.5 0.5 1.0]  GraphicVisPropType=SimpleVisualProperties
  Plates : Subsystem
      mask Display:
      | image(fullfile(matlabroot,'toolbox','physmod','sm','smdemos','backhoe','images','sm_backhoe_mountingplates.png'));
      | port_label('lconn',1,'LA');
      | port_label('lconn',2,'LC');
      | port_label('lconn',3,'AAL');
      | port_label('rconn',1,'B');
      | port_label('rconn',2,'AAR');
  Right Pin : sm_lib/Body Elements/Cylindrical Solid  GraphicAmbientColor=[0.15 0.15 0.15 1.0]  BasedOnType=Density  CenterOfMass=[0 0 0]  CenterOfMassUnits=m  GraphicDiffuseColor=gray  CylinderLength=Tarm*1.2  CylinderLengthUnits=m  CylinderRadius=RH3  CylinderRadiusUnits=m  Density=rhoSteel  DensityUnits=kg/(m^3)  DoExposeReferenceFrame=on  GraphicEmissiveColor=[0.0 0.0 0.0 1.0]  ExportEntireGeometry=off  SerializedFrames=<Frames/>  MarkerShape=Sphere  MarkerSize=10  GraphicType=FromGeometry  InertiaType=CalculateFromGeometry  Mass=1  MassUnits=kg  MomentsOfInertia=[1 1 1]  MomentsOfInertiaUnits=kg*m^2  GraphicOpacity=1.0  ProductsOfInertia=[0 0 0]  ProductsOfInertiaUnits=kg*m^2  GraphicShininess=75  GraphicSpecularColor=[0.5 0.5 0.5 1.0]  GraphicVisPropType=SimpleVisualProperties
  Single Bracket : sm_backhoe_lib/Single Bracket  Hbracket=Lbracket  Wbracket=Dplates-Tplate  Tbracket=Hright  Hhole=Hhole  Rhole=Rhole  Nc=25  bracketColor=orange  rho=rho
      settings: SourceProductBaseCode=MS
  Left Head : PMIOPort  Side=Left
  Right Head : PMIOPort  Port=2  Side=Right
  Cylinder Base : PMIOPort  Port=3  Side=Left
  Lower Arm : PMIOPort  Port=4  Side=Left
  Mounting Base : PMIOPort  Port=5  Side=Right
  connections:
  Lower Arm/RConn1 -- Plates/LConn1
  Plates/LConn2 -- Cylinder Base/RConn1
  Single Bracket/LConn1 -- Plates/RConn1
  Mounting Base/RConn1 -- Single Bracket/RConn1
  Attachment Arm Left/RConn1 -- Plates/LConn3 -- Bracket Transform Left/LConn1
  Left Pin/RConn1 -- Left Head/RConn1 -- Bracket Left/RConn1
  Bracket Transform Left/RConn1 -- Bracket Left/LConn1
  Attachment Arm Right/RConn1 -- Plates/RConn2 -- Bracket Transform Right/LConn1
  Right Head/RConn1 -- Right Pin/RConn1 -- Bracket Right/RConn1
  Bracket Transform Right/RConn1 -- Bracket Right/LConn1
